simulink model "hosmo3_sim"  (R2021b)
settings: Solver=ode8  StartTime=0.0  StopTime=10.0  FixedStep=10^(-4)  RelTol=1e-3
settings Model: Creator=wkw  LastModifiedBy=wkw

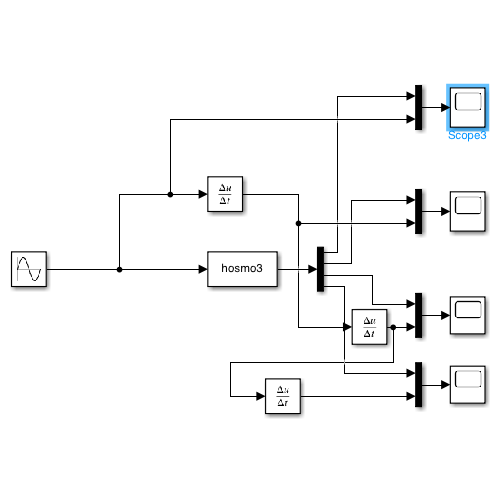
[thumbnail: Simulink's stored preview of the top-level diagram]
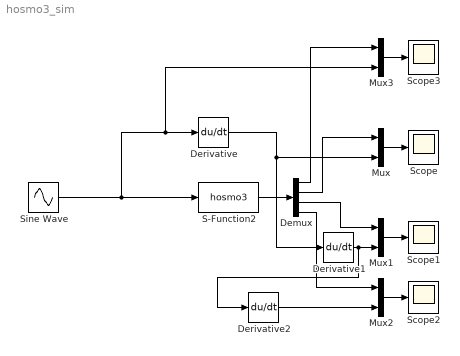
== system hosmo3_sim ==
  Demux : Demux
  Derivative : Derivative
  Derivative1 : Derivative
  Derivative2 : Derivative
  Mux{,1..3} (4 alike) : Mux  Inputs=2
  S-Function2 : S-Function  FunctionName=hosmo3  SFunctionDeploymentMode=off  EnableBusSupport=off
  Scope{,1..3} (4 alike) : Scope
  Sine Wave : Sin  SampleTime=0
  wires:
  Sine Wave/1 -> S-Function2/1, Mux3/2, Derivative/1
  S-Function2/1 -> Demux/1
  Mux1/1 -> Scope1/1
  Demux/3 -> Mux1/1
  Derivative/1 -> Derivative1/1, Mux/2
  Mux/1 -> Scope/1
  Demux/2 -> Mux/1
  Derivative1/1 -> Derivative2/1, Mux1/2
  Derivative2/1 -> Mux2/2
  Demux/4 -> Mux2/1
  Mux2/1 -> Scope2/1
  Mux3/1 -> Scope3/1
  Demux/1 -> Mux3/1
